simulink library "ChimeSignalGeneratorLibBtc"  (R2022b)
settings: Solver=VariableStepAuto  StartTime=0.0  StopTime=10.0  RelTol=1e-3
libraries: simulink x12, dspmathops x3, FeaturePath x1, HandyTextFile x1, RTC x1
(part 2 of 2)

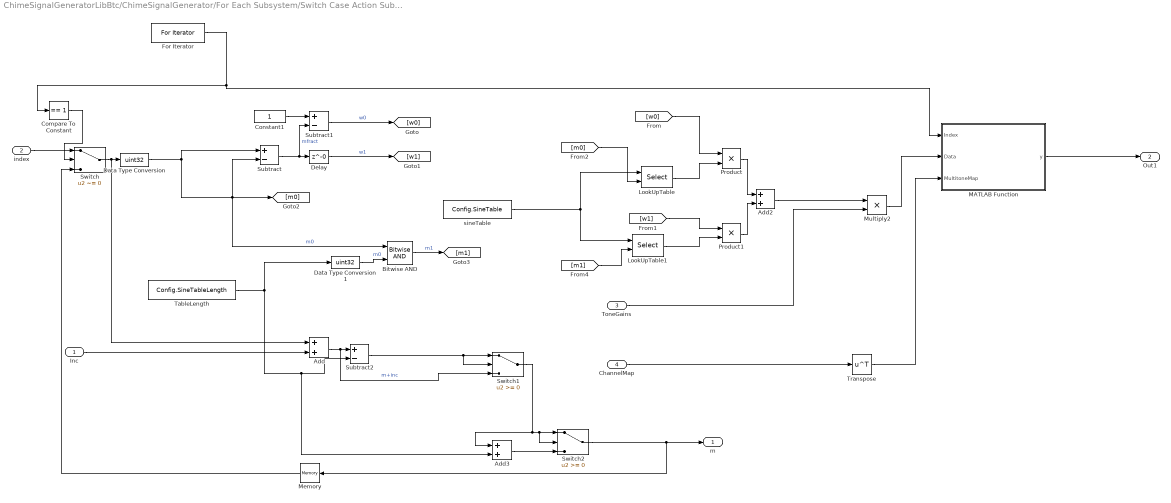
== system ChimeSignalGeneratorLibBtc/ChimeSignalGenerator/For Each Subsystem/Switch Case Action Subsystem5/SigGen_Multitone/Multitone Engine/For Iterator Subsystem ==
  "Inc " : Inport
  index : Inport  Port=2
  ToneGains : Inport  Port=3
  ChannelMap : Inport  Port=4
  Add : Sum
  Add2 : Sum
  Add3 : Sum
  Bitwise AND : simulink/Logic and Bit Operations/Bitwise Operator  logicop=AND  UseBitMask=off  NumInputPorts=2  BitMask=bin2dec('11011001')  BitMaskRealWorld=Stored Integer
  Compare To Constant : simulink/Logic and Bit Operations/Compare To Constant  relop===  const=1  OutDataTypeStr=boolean
  Constant1 : Constant  OutDataTypeStr=single
  Data Type Conversion : DataTypeConversion  OutDataTypeStr=uint32  SaturateOnIntegerOverflow=off  RndMeth=Floor
  Data Type Conversion1 : DataTypeConversion  OutDataTypeStr=uint32  SaturateOnIntegerOverflow=off  RndMeth=Floor
  Delay : Delay  DelayLength=0
  For Iterator : ForIterator  ResetStates=reset  IterationLimit=Config.FrameSizeSamples
  LookUpTable : Selector  IndexMode=Zero-based  InputPortWidth=Config.SineTableLength  IndexOptions=Index vector (port)  Indices=[1 3]  OutputSizes=1
  LookUpTable1 : Selector  IndexMode=Zero-based  InputPortWidth=Config.SineTableLength  IndexOptions=Index vector (port)  Indices=[1 3]  OutputSizes=1
  MATLAB Function : MATLAB Function  TreatAsAtomicUnit=on
  Memory : Memory  InheritSampleTime=on
  Multiply2 : Product
  Product : Product
  Product1 : Product
  Subtract : Sum  Inputs=+-  OutDataTypeStr=single
  Subtract1 : Sum  Inputs=+-  OutDataTypeStr=single
  Subtract2 : Sum  Inputs=+-
  Switch : Switch  Criteria=u2 ~= 0  SaturateOnIntegerOverflow=off  InputSameDT=off
  Switch1 : Switch  SaturateOnIntegerOverflow=off  InputSameDT=off
  Switch2 : Switch  SaturateOnIntegerOverflow=off  InputSameDT=off
  TableLength : Constant  Value=Config.SineTableLength  VectorParams1D=off  OutDataTypeStr=single
  Transpose : Math  Operator=transpose  SignedPower=on
  sineTable : Constant  Value=Config.SineTable  OutDataTypeStr=single
  m : Outport  VectorParamsAs1DForOutWhenUnconnected=off
  Out1 : Outport  Port=2  VectorParamsAs1DForOutWhenUnconnected=off
  wires:
  Transpose/1 -> MATLAB Function/3(MultitoneMap)
  Bitwise AND/1 -> [m1]  "m1"
  Add3/1 -> Switch2/3
  Subtract2/1 -> Switch1/2, Switch1/1
  Switch2/1 -> Memory/1, m/1
  Switch1/1 -> Switch2/1, Switch2/2, Add3/1
  Data Type Conversion1/1 -> Bitwise AND/2  "m0"
  "Inc "/1 -> Add/2
  ToneGains/1 -> Multiply2/2
  MATLAB Function/1(y) -> Out1/1
  Product1/1 -> Add2/2
  Product/1 -> Add2/1
  LookUpTable1/1 -> Product1/2
  [w1] -> Product1/1
  [m1] -> LookUpTable1/2
  LookUpTable/1 -> Product/2
  [w0] -> Product/1
  [m0] -> LookUpTable/2
  sineTable/1 -> LookUpTable1/1, LookUpTable/1
  Delay/1 -> [w1]  "w1"
  Subtract1/1 -> [w0]  "w0"
  Constant1/1 -> Subtract1/1
  Subtract/1 -> Subtract1/2, Delay/1  "mfract"
  Data Type Conversion/1 -> Subtract/1, [m0], Subtract/2, Bitwise AND/1  "m0"
  Memory/1 -> Switch/3
  For Iterator/1 -> Compare To Constant/1, MATLAB Function/1(Index)
  Add/1 -> Subtract2/1, Switch1/3  "m+inc"
  Switch/1 -> Data Type Conversion/1, Add/1
  index/1 -> Switch/1
  Compare To Constant/1 -> Switch/2
  TableLength/1 -> Data Type Conversion1/1, Subtract2/2, Add3/2
  ChannelMap/1 -> Transpose/1
  Multiply2/1 -> MATLAB Function/2(Data)
  Add2/1 -> Multiply2/1

== system ChimeSignalGeneratorLibBtc/ChimeSignalGenerator/For Each Subsystem/Switch Case Action Subsystem/Log Sweep Signal Generator/Log Sweep Engine/Configuration_sublock/  ==
  inc_start_In1 : Inport
  inc_end_In2 : Inport  Port=2
  steps_In3 : Inport  Port=3
  Math Function : Math  Operator=pow  SignedPower=on
  Multiply : Product  Inputs=*/
  Multiply1 : Product  Inputs=*/
  oneVal : Constant  OutDataTypeStr=single
  inc_delta_Out1 : Outport  VectorParamsAs1DForOutWhenUnconnected=off
  wires:
  Multiply1/1 -> Math Function/2
  Multiply/1 -> Math Function/1
  oneVal/1 -> Multiply1/1  "1"
  steps_In3/1 -> Multiply1/2  "steps"
  Math Function/1 -> inc_delta_Out1/1  "inc_delta"
  inc_end_In2/1 -> Multiply/1  "inc_end"
  inc_start_In1/1 -> Multiply/2  "inc_start"

== system ChimeSignalGeneratorLibBtc/ChimeSignalGenerator/For Each Subsystem/Switch Case Action Subsystem1/Linear Sweep Signal Generator/Linear Sweep Engine/Configuration_sublock/  ==
  inc_start_In1 : Inport
  inc_end_In2 : Inport  Port=2
  steps_In3 : Inport  Port=3
  Add : Sum  Inputs=+-
  Multiply1 : Product  Inputs=*/
  inc_delta_Out1 : Outport  VectorParamsAs1DForOutWhenUnconnected=off
  wires:
  inc_start_In1/1 -> Add/2  "inc_start"
  inc_end_In2/1 -> Add/1  "inc_end"
  Add/1 -> Multiply1/1
  Multiply1/1 -> inc_delta_Out1/1
  steps_In3/1 -> Multiply1/2  "steps"

== system ChimeSignalGeneratorLibBtc/ChimeSignalGenerator/For Each Subsystem/Switch Case Action Subsystem2/Old Sweep Signal Generator/Old Sweep Engine/Configuration_sublock/  ==
  inc_start_In1 : Inport
  inc_end_In2 : Inport  Port=2
  steps_In3 : Inport  Port=3
  Add : Sum  Inputs=+-
  Multiply1 : Product  Inputs=*/
  Subtract : Sum  Inputs=+-
  oneVal : Constant  OutDataTypeStr=uint32
  inc_delta_Out1 : Outport  VectorParamsAs1DForOutWhenUnconnected=off
  wires:
  Subtract/1 -> Multiply1/2
  oneVal/1 -> Subtract/2
  steps_In3/1 -> Subtract/1  "steps_state"
  Multiply1/1 -> inc_delta_Out1/1
  Add/1 -> Multiply1/1
  inc_end_In2/1 -> Add/1  "inc_end"
  inc_start_In1/1 -> Add/2  "inc_start"

== matlab function ChimeSignalGeneratorLibBtc/ChimeSignalGenerator/For Each Subsystem/Switch Case Action Subsystem1/Linear Sweep Signal Generator/Linear Sweep Engine/For Iterator Subsystem/MATLAB Function ==
  data: Index input; Data input; y output size=[frameSize_samples, 1]; frameSize_samples parameter
function y = fcn(Index, Data,frameSize_samples)
% comment
Numchannels=1;
y=single(zeros(frameSize_samples,Numchannels));
% init
persistent OutStore ;
if(isempty(OutStore))
    %OutStore = single(size_matrix);
    OutStore =single(zeros(frameSize_samples,Numchannels));
end
% fill out data
OutStore(Index,1:Numchannels) = Data(1,1)';
y = OutStore;

== matlab function ChimeSignalGeneratorLibBtc/ChimeSignalGenerator/For Each Subsystem/Switch Case Action Subsystem/Log Sweep Signal Generator/Log Sweep Engine/For Iterator Subsystem/MATLAB Function ==
  data: Index input; Data input; y output size=[frameSize_samples, 1]; frameSize_samples parameter
function y = fcn(Index, Data,frameSize_samples)
% comment
Numchannels=1;
% init
y=single(zeros(frameSize_samples,Numchannels));
persistent OutStore;
% check if empty
if(isempty(OutStore))
    OutStore =single(zeros(frameSize_samples,Numchannels));
end
% fill out data
OutStore(Index,1:Numchannels) = Data(1,1)';
y = OutStore;

== matlab function ChimeSignalGeneratorLibBtc/ChimeSignalGenerator/For Each Subsystem/Switch Case Action Subsystem2/Old Sweep Signal Generator/Old Sweep Engine/For Iterator Subsystem/MATLAB Function ==
  data: Index input; Data input; y output size=[frameSize_samples, 1]; frameSize_samples parameter
function y = fcn(Index, Data,frameSize_samples)
% comment
Numchannels=1;
y = single(zeros(frameSize_samples,Numchannels));
% init
persistent OutStore ;
if(isempty(OutStore))
    %OutStore = single(size_matrix);
    OutStore = single(zeros(frameSize_samples,Numchannels));
end
% fill out data 
OutStore(Index,1:Numchannels) = Data(1,1)';
y = OutStore;

== matlab function ChimeSignalGeneratorLibBtc/ChimeSignalGenerator/For Each Subsystem/Switch Case Action Subsystem5/SigGen_Multitone/Multitone Engine/For Iterator Subsystem/MATLAB Function ==
  data: Index input; Data input; y output size=[frameSize_samples, 1]; MultitoneMap input; frameSize_samples parameter
function y = fcn(Index,Data,MultitoneMap, frameSize_samples)
% comment
OutChNumSize = 1;
y=single(zeros(frameSize_samples,OutChNumSize));
% init
persistent OutStore ;
if(isempty(OutStore))
    OutStore = single(zeros(frameSize_samples,OutChNumSize));
    
end
for OutChNum = 1:OutChNumSize
    ToneSize = MultitoneMap;
    OutStore(Index,OutChNum) = Data(1,1)+Data(1,2);%Data(1,(OutChNum-1)*ToneSize+1) + Data(1,ToneSize*OutChNum);
end
% fill out data
y = OutStore;

== matlab function ChimeSignalGeneratorLibBtc/ChimeSignalGenerator/For Each Subsystem/Switch Case Action Subsystem3/SigGen_Noise/For Iterator Subsystem/MATLAB Function ==
  data: Index input; Data input; y output size=[frameSize_samples, 1]; frameSize_samples parameter
function y = fcn(Index, Data,frameSize_samples)
% comment
Numchannels = 1;
y=single(zeros(frameSize_samples,Numchannels));
% init
persistent OutStore ;
if(isempty(OutStore))
    %  OutStore = single(size_matrix);
    OutStore = single(zeros(frameSize_samples,Numchannels));
end
% fill out data
OutStore(Index,1:Numchannels) = Data(1,1)';
y = OutStore;

== matlab function ChimeSignalGeneratorLibBtc/ChimeSignalGenerator/For Each Subsystem/Switch Case Action Subsystem4/SigGen_Sawtooth/For Iterator Subsystem/MATLAB Function ==
  data: Index input; Data input; y output size=[frameSize_samples, 1]; frameSize_samples parameter
function y = fcn(Index, Data,frameSize_samples)
% comment
Numchannels = 1;
y=single(zeros(frameSize_samples,Numchannels));
% init
persistent OutStore ;
if(isempty(OutStore))
    % OutStore = single(size_matrix);
    OutStore =single(zeros(frameSize_samples,Numchannels));
end
% fill out data
OutStore(Index,1:Numchannels) = Data(1,1)';
y = OutStore;
